simulink model "Flight_Simulation"  (R2021b)
settings: Solver=ode4  StartTime=0.0  StopTime=20  FixedStep=Settings.Simulation.step_size  RelTol=1e-3  EnableMultiTasking=on
undefined symbols (not defined in the file or in its folder): AeroCoeff, Aircraft, ControlGains, dLEF, Environment, F, Light, MIL, Settings, Trim, trim_control, trim_state, trim_thrust
libraries: simulink x19, simulink_extras x14, slpidlib x2, aerolibfltsims x2, aerolibwind2 x1, vrlib x1
(part 1 of 5)
settings Model: Creator=ole_o  LastModifiedBy=s2051295
settings SolverCC: AlgebraicLoopSolver=TrustRegion
settings DataIOCC: Decimation=50  ExternalInput=U_in  InitialState=[]  LoadExternalInput=on  SaveFormat=StructureWithTime  ReturnWorkspaceOutputs=off  TimeSaveName=t_out  OutputSaveName=X_out, X_dot_out, Y_out  SignalLoggingName=sigsOut
settings OptimizationCC: BooleanDataType=off  DefaultParameterBehavior=Inlined  BufferReuse=off
settings DebuggingCC: UnderspecifiedInitializationDetection=Classic  MergeDetectMultiDrivingBlocksExec=none  SignalResolutionControl=TryResolveAllWithWarning  MultiTaskDSMMsg=warning  MultiTaskCondExecSysMsg=none
settings HardwareCC: ProdBitPerPointer=32  ProdBitPerSizeT=32  ProdBitPerPtrDiffT=32  ProdWordSize=32  ProdHWDeviceType=Intel->x86-32 (Windows32)
settings ModelReferenceCC: PropagateSignalLabelsOutOfModel=off
settings SFSimCC: CustomCodeUndefinedFunction=UseInterfaceOnly

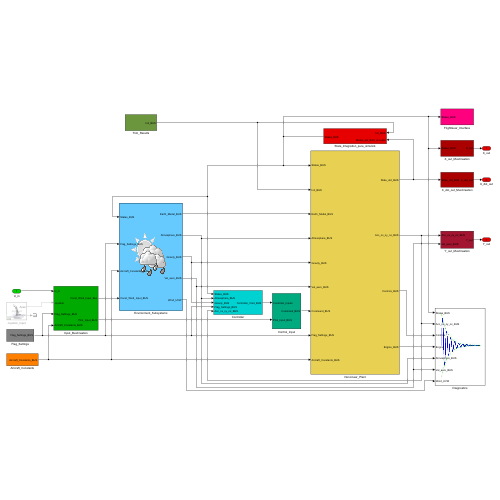
[thumbnail: Simulink's stored preview of the top-level diagram]
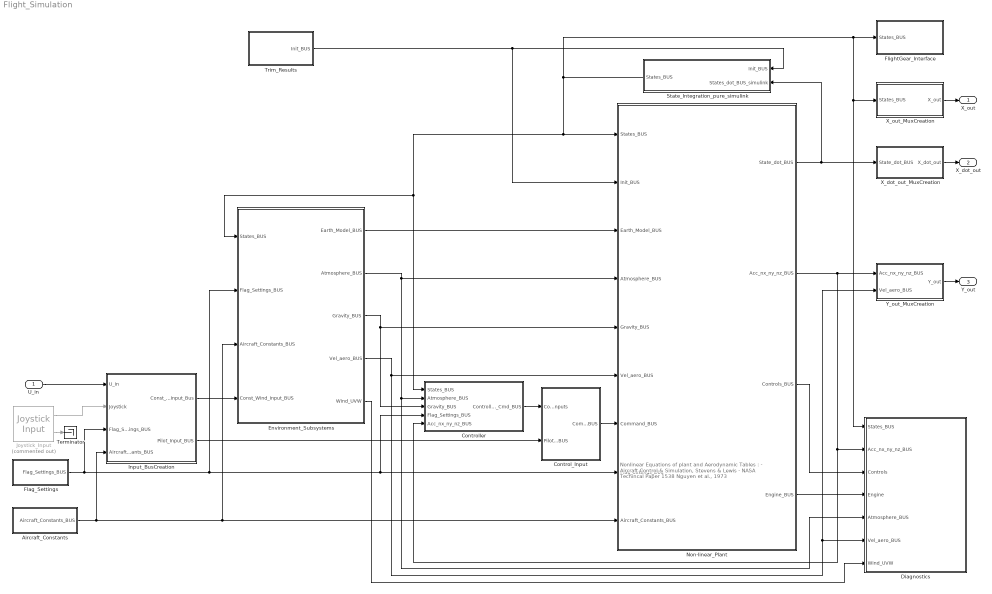
== system Flight_Simulation ==
  note: Nonlinear Equations of plant and Aerodynamic Tables :
      | - Aircraft Control & Simulation, Stevens & Lewis
      | - NASA Techincal Paper 1538 Nguyen et al., 1973
  U_in : Inport  PortDimensions=8
  Aircraft_Constants : Subsystem
  Control_Input : Subsystem
  Controller : Subsystem
  Diagnostics : Subsystem
      mask Display: image('Diagnostics.jpg'); % Use "Edit Image" on toolstrip to change.
  Environment_Subsystems : Subsystem
      mask Display: image('Wetter.jpg'); % Use "Edit Image" on toolstrip to change.
  Flag_Settings : Subsystem
  FlightGear_Interface : Subsystem
  Input_BusCreation : Subsystem
  Joystick_Input : vrlib/Joystick Input  Commented=on  joyid=1  adjustports=off  forcefeed=off
  Non-linear_Plant : Subsystem
  State_Integration_pure_simulink : Subsystem
  Terminator : Terminator
  Trim_Results : Subsystem
  X_dot_out_MuxCreation : Subsystem
  X_out_MuxCreation : Subsystem
  Y_out_MuxCreation : Subsystem
  X_out : Outport
  X_dot_out : Outport  Port=2
  Y_out : Outport  Port=3
  wires:
  Non-linear_Plant/4(Engine_BUS) -> Diagnostics/4(Engine)
  Input_BusCreation/1(Const_Wind_Input_Bus) -> Environment_Subsystems/4(Const_Wind_Input_BUS)
  Joystick_Input/2 -> Terminator/1
  Non-linear_Plant/3(Controls_BUS) -> Diagnostics/3(Controls)
  Environment_Subsystems/3(Gravity_BUS) -> Non-linear_Plant/5(Gravity_BUS), Controller/3(Gravity_BUS)
  Joystick_Input/1 -> Input_BusCreation/2(Joystick)
  Aircraft_Constants/1(Aircraft_Constants_BUS) -> Environment_Subsystems/3(Aircraft_Constants_BUS), Non-linear_Plant/9(Aircraft_Constants_BUS), Input_BusCreation/4(Aircraft_Constants_BUS)
  X_out_MuxCreation/1(X_out) -> X_out/1
  Environment_Subsystems/4(Vel_aero_BUS) -> Non-linear_Plant/6(Vel_aero_BUS), Diagnostics/6(Vel_aero_BUS), Y_out_MuxCreation/2(Vel_aero_BUS)
  Controller/1(Controller_Cmd_BUS) -> Control_Input/1(Controller_Inputs)
  Environment_Subsystems/2(Atmosphere_BUS) -> Non-linear_Plant/4(Atmosphere_BUS), Diagnostics/5(Atmosphere_BUS), Controller/2(Atmosphere_BUS)
  State_Integration_pure_simulink/1(States_BUS) -> FlightGear_Interface/1(States_BUS), X_out_MuxCreation/1(States_BUS), Diagnostics/1(States_BUS), Non-linear_Plant/1(States_BUS), Environment_Subsystems/1(States_BUS), Controller/1(States_BUS)
  Y_out_MuxCreation/1(Y_out) -> Y_out/1
  Input_BusCreation/2(Pilot_Input_BUS) -> Control_Input/2(Pilot_Input_BUS)
  Trim_Results/1(Init_BUS) -> Non-linear_Plant/2(Init_BUS), State_Integration_pure_simulink/1(Init_BUS)
  Control_Input/1(Command_BUS) -> Non-linear_Plant/7(Command_BUS)
  X_dot_out_MuxCreation/1(X_dot_out) -> X_dot_out/1
  Flag_Settings/1(Flag_Settings_BUS) -> Environment_Subsystems/2(Flag_Settings_BUS), Non-linear_Plant/8(Flag_Settings_BUS), Controller/4(Flag_Settings_BUS), Input_BusCreation/3(Flag_Settings_BUS)
  U_in/1 -> Input_BusCreation/1(U_in)
  Non-linear_Plant/1(State_dot_BUS) -> X_dot_out_MuxCreation/1(State_dot_BUS), State_Integration_pure_simulink/2(States_dot_BUS_simulink)
  Non-linear_Plant/2(Acc_nx_ny_nz_BUS) -> Y_out_MuxCreation/1(Acc_nx_ny_nz_BUS), Controller/5(Acc_nx_ny_nz_BUS), Diagnostics/2(Acc_nx_ny_nz_BUS)
  Environment_Subsystems/1(Earth_Model_BUS) -> Non-linear_Plant/3(Earth_Model_BUS)
  Environment_Subsystems/5(Wind_UVW) -> Diagnostics/7(Wind_UVW)

== system Flight_Simulation/Aircraft_Constants ==
  Bus Creator : BusCreator  Inputs=8
  CG_Reference_Location : Subsystem
  Constant : Constant  Value=Aircraft.LandingGearFlg
  Constant1 : Constant  Value=Aircraft.Flaps_degrees
  Constant2 : Constant  Value=Aircraft.F_g.final
  Control_Surface_Model : Subsystem
  Engine_Const : Subsystem
  Mass_Properties : Subsystem
  Wing_Dimensions : Subsystem
  Aircraft_Constants_BUS : Outport
  wires:
  Mass_Properties/1(Mass_Properties_BUS) -> Bus Creator/1
  Wing_Dimensions/1(Wing_Dimension_BUS) -> CG_Reference_Location/1(Wing_Dimension_BUS), Bus Creator/2
  CG_Reference_Location/1(CG_BUS) -> Bus Creator/3
  Engine_Const/1(Engine_Const_BUS) -> Bus Creator/5
  Control_Surface_Model/1(Control_Surface_Const_BUS) -> Bus Creator/4
  Bus Creator/1 -> Aircraft_Constants_BUS/1  "Aircraft_Constants_BUS"
  Constant/1 -> Bus Creator/6  "LandingGearFlg"
  Constant1/1 -> Bus Creator/7  "Flaps_degrees"
  Constant2/1 -> Bus Creator/8  "FlightProfileAlleviationFactor_Fg"

== system Flight_Simulation/Control_Input ==
  Controller_Inputs : Inport
  Pilot_Input_BUS : Inport  Port=2
  Aileron Disturbance : Subsystem
  Bus Creator : BusCreator  Inputs=5
  Bus Selector : BusSelector  OutputSignals=Thrust_N_ctrl,Elevator_deg_ctrl,Aileron_deg_ctrl,Rudder_deg_ctrl,Speedbrakes_%_ctrl
  Bus Selector1 : BusSelector  OutputSignals=Thrust_in_N,Elevator_in_deg,Aileron_in_deg,Rudder_in_deg,Speedbrakes_in_%
  Elevator Disturbance : Subsystem
  Rudder Disturbance : Subsystem
  Sum1 : Sum  Inputs=+++  InputSameDT=on  SaturateOnIntegerOverflow=on  OutDataTypeStr=Inherit: Same as first input
  Sum2 : Sum  Inputs=+++  InputSameDT=on  SaturateOnIntegerOverflow=on  OutDataTypeStr=Inherit: Same as first input
  Sum3 : Sum  Inputs=+++  InputSameDT=on  SaturateOnIntegerOverflow=on  OutDataTypeStr=Inherit: Same as first input
  Sum4 : Sum  Inputs=++|  InputSameDT=on  SaturateOnIntegerOverflow=on  OutDataTypeStr=Inherit: Same as first input
  Sum5 : Sum  Inputs=++|  InputSameDT=on  SaturateOnIntegerOverflow=on  OutDataTypeStr=Inherit: Same as first input
  Command_BUS : Outport
  wires:
  Sum4/1 -> Bus Creator/1  "Thrust_cmd_N"
  Bus Selector/3 -> Sum2/1  "<Aileron_deg_ctrl>"
  Bus Selector/2 -> Sum1/1  "<Elevator_deg_ctrl>"
  Bus Selector/4 -> Sum3/1  "<Rudder_deg_ctrl>"
  Bus Creator/1 -> Command_BUS/1  "Command_BUS"
  Sum1/1 -> Bus Creator/2  "Elevator_cmd_deg"
  Sum2/1 -> Bus Creator/3  "Aileron_cmd_deg"
  Sum3/1 -> Bus Creator/4  "Rudder_cmd_deg"
  Controller_Inputs/1 -> Bus Selector/1
  Bus Selector/1 -> Sum4/1  "<Thrust_N_ctrl>"
  Rudder Disturbance/1(Rudder_Disturbance) -> Sum3/3
  Aileron Disturbance/1(Aileron_Disturbance) -> Sum2/3
  Elevator Disturbance/1(Elevator_Disturbance) -> Sum1/3
  Pilot_Input_BUS/1 -> Bus Selector1/1
  Bus Selector1/1 -> Sum4/2  "<Thrust_in_N>"
  Bus Selector1/2 -> Sum1/2  "<Elevator_in_deg>"
  Bus Selector1/3 -> Sum2/2  "<Aileron_in_deg>"
  Bus Selector1/4 -> Sum3/2  "<Rudder_in_deg>"
  Bus Selector1/5 -> Sum5/2  "<Speedbrakes_in_%>"
  Bus Selector/5 -> Sum5/1  "<Speedbrakes_%_ctrl>"
  Sum5/1 -> Bus Creator/5  "Speedbrakes_cmd_%"

== system Flight_Simulation/Controller ==
  note: must not change name and location
      | - would interfere with TrimAndLin
  States_BUS : Inport
  Atmosphere_BUS : Inport  Port=2
  Gravity_BUS : Inport  Port=3
  Flag_Settings_BUS : Inport  Port=4
  Acc_nx_ny_nz_BUS : Inport  Port=5
  Autopilot : Subsystem
  Bus Creator : BusCreator  Inputs=5
  Bus Selector : BusSelector  OutputSignals=Linearization_Flag,Trim_Flag
  Bypass for TrimAndLin : Switch  Criteria=u2 > Threshold
  Constant{,1..5} (6 alike) : Constant  Value=0
  Logical Operator : Logic  Operator=NOR  AllPortsSameDT=off  OutDataTypeStr=boolean
  Step : Step  Time=0.2  Before=-10  After=0  SampleTime=0
  Terminator : Terminator
  Controller_Cmd_BUS : Outport
  wires:
  States_BUS/1 -> Autopilot/3(States_BUS)
  Constant5/1 -> Bus Creator/2  "Elevator_deg_ctrl"
  Constant/1 -> Bus Creator/1  "Thrust_N_ctrl"
  Constant2/1 -> Bus Creator/3  "Aileron_deg_ctrl"
  Constant3/1 -> Bus Creator/4  "Rudder_deg_ctrl"
  Bus Creator/1 -> Controller_Cmd_BUS/1  "Controller_Cmd_BUS"
  Autopilot/1(d_E) -> Bypass for TrimAndLin/1
  Flag_Settings_BUS/1 -> Bus Selector/1
  Bus Selector/1 -> Logical Operator/1  "<Linearization_Flag>"
  Bus Selector/2 -> Logical Operator/2  "<Trim_Flag>"
  Logical Operator/1 -> Bypass for TrimAndLin/2
  Constant1/1 -> Bypass for TrimAndLin/3  "d_Ec"
  Constant4/1 -> Bus Creator/5  "Speedbrakes_%_ctrl"
  Acc_nx_ny_nz_BUS/1 -> Terminator/1
  Gravity_BUS/1 -> Autopilot/1(Gravity_BUS)
  Atmosphere_BUS/1 -> Autopilot/2(Atmosphere_BUS)

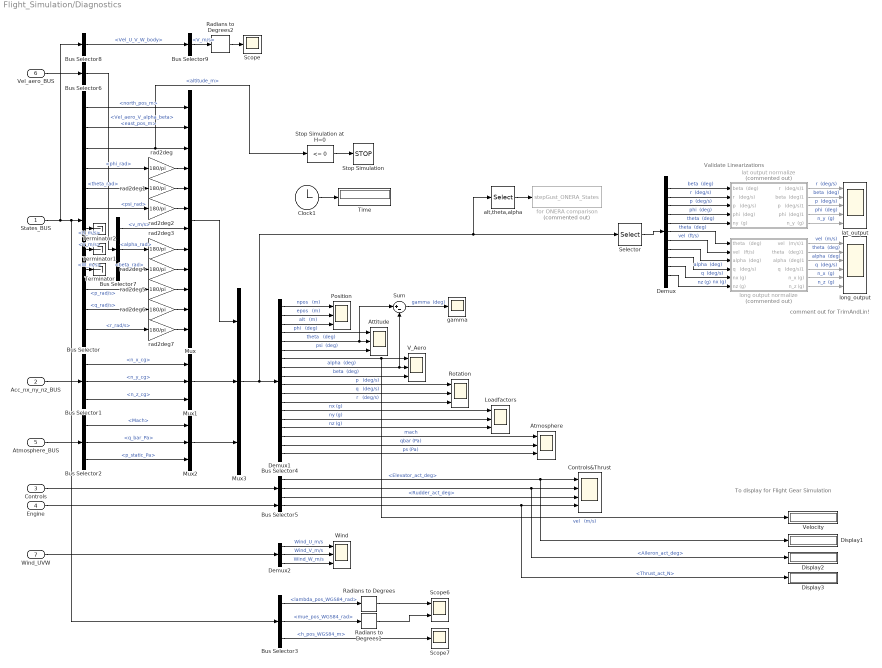
== system Flight_Simulation/Diagnostics ==
  note: To display for
      | Flight Gear Simulation
  note: comment out for TrimAndLin!
  note: Validate Linearizations
  States_BUS : Inport
  Acc_nx_ny_nz_BUS : Inport  Port=2
  Controls : Inport  Port=3
  Engine : Inport  Port=4
  Atmosphere_BUS : Inport  Port=5
  Vel_aero_BUS : Inport  Port=6
  Wind_UVW : Inport  Port=7
  Atmosphere : Scope  NumInputPorts=3
  Attitude : Scope  NumInputPorts=3
  Bus Selector : BusSelector  OutputSignals=Position_north_east_alt.north_pos_m,Position_north_east_alt.east_pos_m,Position_north_east_alt.altitude_m,Angles_phi_theta_psi.phi_rad,Angles_phi_theta_psi.theta_rad,Angles_phi_theta_psi.psi_rad,Vel_U_V_W_body.U_m/s,Vel_U_V_W_body.V_m/s,Vel_U_V_W_body.W_m/s,Rates_p_q_r.p_rad/s,Rates_p_q_r.q_rad/s,Rates_p_q_r.r_rad/s
  Bus Selector1 : BusSelector  OutputSignals=n_x_cg,n_y_cg,n_z_cg
  Bus Selector2 : BusSelector  OutputSignals=Mach,q_bar_Pa,p_static_Pa
  Bus Selector3 : BusSelector  OutputSignals=Pos_WGS84.lambda_pos_WGS84_rad,Pos_WGS84.mue_pos_WGS84_rad,Pos_WGS84.h_pos_WGS84_m
  Bus Selector4 : BusSelector  OutputSignals=Elevator_act_deg,Aileron_act_deg,Rudder_act_deg
  Bus Selector5 : BusSelector  OutputSignals=Thrust_act_N
  Bus Selector6 : BusSelector  OutputSignals=Vel_aero_V_alpha_beta
  Bus Selector7 : BusSelector  OutputSignals=v_m/s,alpha_rad,beta_rad
  Bus Selector8 : BusSelector  OutputSignals=Vel_U_V_W_body
  Bus Selector9 : BusSelector  OutputSignals=V_m/s
  Clock1 : Clock
  Controls&Thrust : Scope  NumInputPorts=4
  Demux : Demux  Outputs=11
  Demux1 : Demux  Outputs=18
      settings: DisplayOption=none
  Demux2 : Demux  Outputs=3
  Display1 : Display
  Display2 : Display
  Display3 : Display
  Loadfactors : Scope  NumInputPorts=3
  Mux : Mux  Inputs=12
  Mux1 : Mux  Inputs=3
  Mux2 : Mux  Inputs=3
  Mux3 : Mux  Inputs=3
  Position : Scope  NumInputPorts=3
  Radians to Degrees : simulink_extras/Transformations/Radians to Degrees
  Radians to Degrees1 : simulink_extras/Transformations/Radians to Degrees
  Radians to Degrees2 : simulink_extras/Transformations/Radians to Degrees
  Rotation : Scope  NumInputPorts=3
  Scope : Scope
  Scope6 : Scope  NumInputPorts=2
  Scope7 : Scope
  Selector : Selector  InputPortWidth=18  IndexOptions=Index vector (dialog)  Indices=[9 12 10 4 14 5 7 8 11 13 15]  OutputSizes=1
  Stop Simulation : Stop
  Stop Simulation at H=0 : simulink/Logic and Bit Operations/Compare To Constant  relop=<=  const=0  OutDataTypeStr=boolean
  Sum : Sum  Inputs=|+-
  Terminator : Terminator
  Terminator1 : Terminator
  Terminator2 : Terminator
  Time : Display
  V_Aero : Scope  NumInputPorts=3
  Velocity : Display
  Wind : Scope  NumInputPorts=3
  alt,theta,alpha : Selector  InputPortWidth=18  IndexOptions=Index vector (dialog)  Indices=[3 5 8]  OutputSizes=1
  for ONERA comparison : ToWorkspace  Commented=on  VariableName=stepGust_ONERA_States  SampleTime=-1
  gamma : Scope
  lat output normalize : Subsystem  Commented=on
  lat_output : Scope  NumInputPorts=5
  long output normalize : Subsystem  Commented=on
  long_output : Scope  NumInputPorts=6
  rad2deg{,1..7} (8 alike) : Gain  Gain=180/pi
  wires:
  Demux1/1 -> Position/1  "npos   (m)"
  Demux1/2 -> Position/2  "epos   (m)"
  Demux1/3 -> Position/3  "alt   (m)"
  Demux1/5 -> Attitude/2, Sum/1  "theta   (deg)"
  Demux1/6 -> Attitude/3  "psi  (deg)"
  Demux1/7 -> V_Aero/1, Velocity/1  "vel   (m/s)"
  Demux1/9 -> V_Aero/3  "beta  (deg)"
  Demux1/10 -> Rotation/1  "p   (deg/s)"
  Demux1/11 -> Rotation/2  "q   (deg/s)"
  Demux1/12 -> Rotation/3  "r   (deg/s)"
  Demux1/13 -> Loadfactors/1  "nx (g)"
  Demux1/14 -> Loadfactors/2  "ny (g)"
  Demux1/15 -> Loadfactors/3  "nz (g)"
  Demux1/4 -> Attitude/1  "phi   (deg)"
  Demux1/16 -> Atmosphere/1  "mach"
  Demux1/17 -> Atmosphere/2  "qbar (Pa)"
  Demux1/18 -> Atmosphere/3  "ps (Pa)"
  States_BUS/1 -> Bus Selector8/1, Bus Selector3/1, Bus Selector/1
  Bus Selector/1 -> Mux/1  "<north_pos_m>"
  Bus Selector/2 -> Mux/2  "<east_pos_m>"
  Bus Selector/11 -> rad2deg6/1  "<q_rad/s>"
  Bus Selector/10 -> rad2deg5/1  "<p_rad/s>"
  Bus Selector/12 -> rad2deg7/1  "<r_rad/s>"
  Bus Selector/4 -> rad2deg/1  "<phi_rad>"
  Bus Selector/3 -> Stop Simulation at H=0/1, Mux/3  "<altitude_m>"
  Bus Selector/5 -> rad2deg1/1  "<theta_rad>"
  Bus Selector/6 -> rad2deg2/1  "<psi_rad>"
  rad2deg/1 -> Mux/4
  rad2deg1/1 -> Mux/5
  rad2deg2/1 -> Mux/6
  rad2deg3/1 -> Mux/8
  rad2deg4/1 -> Mux/9
  rad2deg5/1 -> Mux/10
  rad2deg6/1 -> Mux/11
  rad2deg7/1 -> Mux/12
  Mux/1 -> Mux3/1
  Acc_nx_ny_nz_BUS/1 -> Bus Selector1/1
  Bus Selector1/2 -> Mux1/2  "<n_y_cg>"
  Bus Selector1/1 -> Mux1/1  "<n_x_cg>"
  Bus Selector1/3 -> Mux1/3  "<n_z_cg>"
  Atmosphere_BUS/1 -> Bus Selector2/1
  Bus Selector2/3 -> Mux2/3  "<p_static_Pa>"
  Bus Selector2/2 -> Mux2/2  "<q_bar_Pa>"
  Bus Selector2/1 -> Mux2/1  "<Mach>"
  Mux2/1 -> Mux3/3
  Mux1/1 -> Mux3/2
  Mux3/1 -> alt,theta,alpha/1, Selector/1, Demux1/1
  Bus Selector3/1 -> Radians to Degrees/1  "<lambda_pos_WGS84_rad>"
  Bus Selector3/2 -> Radians to Degrees1/1  "<mue_pos_WGS84_rad>"
  Bus Selector3/3 -> Scope7/1  "<h_pos_WGS84_m>"
  Radians to Degrees1/1 -> Scope6/2
  Radians to Degrees/1 -> Scope6/1
  Clock1/1 -> Time/1
  long output normalize/1(vel   (m/s)1) -> long_output/1  "vel  (m/s)"
  long output normalize/2(theta   (deg)1) -> long_output/2  "theta  (deg)"
  long output normalize/3(alpha  (deg)1) -> long_output/3  "alpha  (deg)"
  long output normalize/6(n_z (g)) -> long_output/6  "n_z  (g)"
  Sum/1 -> gamma/1  "gamma  (deg)"
  Demux1/8 -> V_Aero/2, Sum/2  "alpha  (deg)"
  Controls/1 -> Bus Selector4/1
  Bus Selector4/1 -> Display1/1, Controls&Thrust/1  "<Elevator_act_deg>"
  Bus Selector4/2 -> Display2/1, Controls&Thrust/2  "<Aileron_act_deg>"
  Bus Selector5/1 -> Controls&Thrust/4, Display3/1  "<Thrust_act_N>"
  Engine/1 -> Bus Selector5/1
  long output normalize/4(q   (deg/s)1) -> long_output/4  "q  (deg/s)"
  lat output normalize/2(beta  (deg)1) -> lat_output/2  "beta  (deg)"
  lat output normalize/1(r   (deg/s)1) -> lat_output/1  "r  (deg/s)"
  lat output normalize/3(p   (deg/s)1) -> lat_output/3  "p  (deg/s)"
  lat output normalize/4(phi  (deg)1) -> lat_output/4  "phi  (deg)"
  Selector/1 -> Demux/1
  Demux/2 -> lat output normalize/2(r   (deg/s))  "r  (deg/s)"
  Demux/3 -> lat output normalize/3(p   (deg/s))  "p  (deg/s)"
  Demux/4 -> lat output normalize/4(phi  (deg))  "phi  (deg)"
  Demux/6 -> long output normalize/1(theta   (deg))  "theta  (deg)"
  Demux/7 -> long output normalize/2(vel   (ft/s))  "vel  (ft/s)"
  Demux/8 -> long output normalize/3(alpha  (deg))  "alpha  (deg)"
  Demux/9 -> long output normalize/4(q   (deg/s))  "q  (deg/s)"
  Demux/11 -> long output normalize/6(nz (g))  "nz (g)"
  Demux/1 -> lat output normalize/1(beta  (deg))  "beta  (deg)"
  Bus Selector4/3 -> Controls&Thrust/3  "<Rudder_act_deg>"
  Stop Simulation at H=0/1 -> Stop Simulation/1
  Wind_UVW/1 -> Demux2/1
  Demux2/1 -> Wind/1  "Wind_U_m/s"
  Demux2/2 -> Wind/2  "Wind_V_m/s"
  Demux2/3 -> Wind/3  "Wind_W_m/s"
  alt,theta,alpha/1 -> for ONERA comparison/1
  Vel_aero_BUS/1 -> Bus Selector6/1
  Bus Selector6/1 -> Bus Selector7/1  "<Vel_aero_V_alpha_beta>"
  Bus Selector7/2 -> rad2deg3/1  "<alpha_rad>"
  Bus Selector7/3 -> rad2deg4/1  "<beta_rad>"
  Demux/10 -> long output normalize/5(nx (g))  "nx (g)"
  long output normalize/5(n_x (g)) -> long_output/5  "n_x  (g)"
  Demux/5 -> lat output normalize/5(ny  (g))  "theta  (deg)"
  lat output normalize/5(n_y  (g)) -> lat_output/5  "n_y  (g)"
  Bus Selector7/1 -> Mux/7  "<v_m/s>"
  Bus Selector/9 -> Terminator/1  "<W_m/s>"
  Bus Selector/7 -> Terminator2/1  "<U_m/s>"
  Bus Selector/8 -> Terminator1/1  "<V_m/s>"
  Bus Selector8/1 -> Bus Selector9/1  "<Vel_U_V_W_body>"
  Bus Selector9/1 -> Radians to Degrees2/1  "<V_m/s>"
  Radians to Degrees2/1 -> Scope/1

== system Flight_Simulation/Environment_Subsystems ==
  note: more efficient
  note: must not change name and location
      | - would interfere with TrimAndLin
  States_BUS : Inport
  Flag_Settings_BUS : Inport  Port=2
  Aircraft_Constants_BUS : Inport  Port=3
  Const_Wind_Input_BUS : Inport  Port=4
  Earth_Model : Subsystem
  Gravity_Model_simple : Subsystem
  ISA_StandardAtmosphere_Model_ScriptVersion : Subsystem
  ISA_StandardAtmosphere_Model_SimulinkVersion : Subsystem
  Manual Switch : ManualSwitch
  Wind_Input : Subsystem
  Wind_Model : Subsystem
  Earth_Model_BUS : Outport
  Atmosphere_BUS : Outport  Port=2
  Gravity_BUS : Outport  Port=3
  Vel_aero_BUS : Outport  Port=4
  Wind_UVW : Outport  Port=5
  wires:
  Gravity_Model_simple/1(Gravity_BUS) -> ISA_StandardAtmosphere_Model_SimulinkVersion/2(Gravity_BUS), ISA_StandardAtmosphere_Model_ScriptVersion/2(Gravity_BUS), Gravity_BUS/1
  Earth_Model/1(Earth_Model_BUS) -> Earth_Model_BUS/1
  Aircraft_Constants_BUS/1 -> Wind_Model/3(Aircraft_Constants_BUS)
  States_BUS/1 -> Wind_Model/2(States_BUS), Wind_Input/1(States_BUS), ISA_StandardAtmosphere_Model_SimulinkVersion/1(States_BUS), ISA_StandardAtmosphere_Model_ScriptVersion/1(States_BUS), Gravity_Model_simple/1(States_BUS), Earth_Model/1(States_BUS)
  ISA_StandardAtmosphere_Model_ScriptVersion/1(Atmosphere_BUS) -> Manual Switch/1
  ISA_StandardAtmosphere_Model_SimulinkVersion/1(Atmosphere_BUS) -> Manual Switch/2
  Manual Switch/1 -> Atmosphere_BUS/1, Wind_Model/1(Atmosphere_BUS)  "Atmosphere_BUS"
  Wind_Model/1(Wind_BUS) -> Wind_UVW/1, Wind_Input/2(Wind_BUS)  "Wind_Vel_UVWe_m/s"
  Const_Wind_Input_BUS/1 -> Wind_Input/4(Const_Wind_Vel_UVWe_m/s)  "Const_Wind_Vel_UVWe_m/s"
  Flag_Settings_BUS/1 -> Wind_Input/3(Flag_Settings_BUS)  "Flag_Settings_BUS"
  Wind_Input/1(Vel_aero_BUS) -> ISA_StandardAtmosphere_Model_SimulinkVersion/3(Vel_aero_BUS), ISA_StandardAtmosphere_Model_ScriptVersion/3(Vel_Aero_BUS), Vel_aero_BUS/1

== system Flight_Simulation/Flag_Settings ==
  Bus Creator : BusCreator  Inputs=3
  Fidelity_Flag : Constant  Value=0
  Lin_Flag : Constant  Value=0
  Trim_Flag : Constant  Value=0
  Flag_Settings_BUS : Outport
  wires:
  Fidelity_Flag/1 -> Bus Creator/1  "Fidelity_Flag"
  Bus Creator/1 -> Flag_Settings_BUS/1  "Flag_Settings_BUS"
  Lin_Flag/1 -> Bus Creator/2  "Linearization_Flag"
  Trim_Flag/1 -> Bus Creator/3  "Trim_Flag"

== system Flight_Simulation/FlightGear_Interface ==
  note: Remark: Set correct Flight Gear installation path
  note: don't rename
      | or IP-address cannot automatically be set
  States_BUS : Inport
  Bus Selector2 : BusSelector  OutputSignals=Angles_phi_theta_psi
  Bus Selector3 : BusSelector  OutputSignals=phi_rad,theta_rad,psi_rad
  Bus Selector4 : BusSelector  OutputSignals=Pos_WGS84
  Bus Selector5 : BusSelector  OutputSignals=lambda_pos_WGS84_rad,mue_pos_WGS84_rad,h_pos_WGS84_m
  Display : Display
  Display1 : Display
  Display2 : Display
  FG_simpleInterface : aerolibfltsims/FlightGear Preconfigured 6DoF Animation  Commented=on  xFlightGearVersion=v2019.1  DestinationIpAddress=192.168.0.166  DestinationPort=5502  SampleTime=-1  packetVersion=24
  GenerateRunScript : aerolibfltsims/Generate Run Script  Architecture=Win64  dataFlow=Receive  GeometryModelName=c172p  AirportId=EDDC  RunwayId=22  InitialAltitude=15000  InitialHeading=113  OffsetDistance=4.72  OffsetAzimuth=0  InstallScenery=on  DisableShaders=off  OriginAddress=127.0.0.1  DestinationPort=5502  OriginPort=5502  LocalAddress=192.168.0.166  OutputFileName=runfg.bat  FlightGearBaseDirectory=D:\FlightGear 2020.3
  Mux1 : Mux  Inputs=6
  Radians to Degrees : simulink_extras/Transformations/Radians to Degrees
  Radians to Degrees1 : simulink_extras/Transformations/Radians to Degrees
  wires:
  States_BUS/1 -> Bus Selector2/1, Bus Selector4/1
  Bus Selector2/1 -> Bus Selector3/1  "<Angles_phi_theta_psi>"
  Bus Selector3/1 -> Mux1/4  "<phi_rad>"
  Bus Selector3/2 -> Mux1/5  "<theta_rad>"
  Bus Selector3/3 -> Mux1/6  "<psi_rad>"
  Mux1/1 -> FG_simpleInterface/1
  Bus Selector4/1 -> Bus Selector5/1  "<Pos_WGS84>"
  Bus Selector5/1 -> Radians to Degrees/1  "<lambda_pos_WGS84_rad>"
  Bus Selector5/2 -> Radians to Degrees1/1  "<mue_pos_WGS84_rad>"
  Bus Selector5/3 -> Display2/1, Mux1/3  "<h_pos_WGS84_m>"
  Radians to Degrees/1 -> Mux1/1, Display/1
  Radians to Degrees1/1 -> Display1/1, Mux1/2

== system Flight_Simulation/Input_BusCreation ==
  U_in : Inport
  Joystick : Inport  Port=2
  Flag_Settings_BUS : Inport  Port=3
  Aircraft_Constants_BUS : Inport  Port=4
  Aileron : Display
  Bus Creator : BusCreator  Inputs=3
  Bus Creator1 : BusCreator  Inputs=5
  Demux : Demux  Outputs=8
  Elevator : Display
  Evaluate Joystick Input : Subsystem
  JS_Aileron : Display
  JS_Elevator : Display
  JS_Thrust : Display
  Manual Switch : ManualSwitch  CurrentSetting=0
  Sum : Sum  Inputs=++|
  Sum1 : Sum  Inputs=++|
  Thrust : Display
  Const_Wind_Input_Bus : Outport
  Pilot_Input_BUS : Outport  Port=2
  wires:
  U_in/1 -> Demux/1
  Evaluate Joystick Input/3(Joystick_Thrust_N) -> Manual Switch/1, JS_Thrust/1  "Thrust_in_N"
  Sum1/1 -> Aileron/1, Bus Creator1/3  "Aileron_in_deg"
  Bus Creator1/1 -> Pilot_Input_BUS/1  "Pilot_Input_BUS"
  Demux/4 -> Bus Creator1/4  "Rudder_in_deg"
  Sum/1 -> Elevator/1, Bus Creator1/2  "Elevator_in_deg"
  Demux/6 -> Bus Creator/1  "const_u_wind_m/s"
  Bus Creator/1 -> Const_Wind_Input_Bus/1  "Wind_Vel_UVW_m/s"
  Demux/7 -> Bus Creator/2  "const_v_wind_m/s"
  Demux/8 -> Bus Creator/3  "const_w_wind_m/s"
  Aircraft_Constants_BUS/1 -> Evaluate Joystick Input/1(Aircraft_Constants_BUS)
  Flag_Settings_BUS/1 -> Evaluate Joystick Input/2(Flag_Settings_BUS)
  Joystick/1 -> Evaluate Joystick Input/3(Joystick)
  Evaluate Joystick Input/1(Joystick_Aileron_deg) -> Sum1/1, JS_Aileron/1
  Evaluate Joystick Input/2(Joystick_Elevator_deg) -> Sum/1, JS_Elevator/1
  Demux/2 -> Sum/2  "Elevator_in_deg"
  Demux/3 -> Sum1/2  "Aileron_in_deg"
  Manual Switch/1 -> Thrust/1, Bus Creator1/1  "Thrust_in_N"
  Demux/1 -> Manual Switch/2  "Thrust_in_N"
  Demux/5 -> Bus Creator1/5  "Speedbrakes_in_%"

== system Flight_Simulation/Non-linear_Plant ==
  States_BUS : Inport
  Init_BUS : Inport  Port=2
  Earth_Model_BUS : Inport  Port=3
  Atmosphere_BUS : Inport  Port=4
  Gravity_BUS : Inport  Port=5
  Vel_aero_BUS : Inport  Port=6
  Command_BUS : Inport  Port=7
  Flag_Settings_BUS : Inport  Port=8
  Aircraft_Constants_BUS : Inport  Port=9
  6DOF_Equations : Subsystem
      mask Display: image('Flightdynamics.png'); % Use "Edit Image" on toolstrip to change.
  Actuator_Models : Subsystem
  Aerodynamic_Modul : Subsystem
  Engine_Model : Subsystem
  State_dot_BUS : Outport
  Acc_nx_ny_nz_BUS : Outport  Port=2
  Controls_BUS : Outport  Port=3
  Engine_BUS : Outport  Port=4
  wires:
  Flag_Settings_BUS/1 -> Engine_Model/2(Flag_Settings_BUS), Actuator_Models/3(Flag_Settings_BUS)
  Command_BUS/1 -> Engine_Model/1(Command_BUS), Actuator_Models/2(Command_BUS)
  Aircraft_Constants_BUS/1 -> Aerodynamic_Modul/4(Aircraft_Constant_BUS), Actuator_Models/5(Aircraft_Constants_BUS), Engine_Model/4(Aircraft_Constants_BUS), 6DOF_Equations/5(Aircraft_Constants_BUS)
  Engine_Model/1(Engine_BUS) -> Engine_BUS/1, Aerodynamic_Modul/7(Engine_BUS), 6DOF_Equations/4(Engine_BUS)
  Atmosphere_BUS/1 -> Engine_Model/5(Atmosphere_BUS), Actuator_Models/6(Atmosphere_BUS), Aerodynamic_Modul/1(Atmosphere_BUS)
  Gravity_BUS/1 -> 6DOF_Equations/6(Gravity_BUS)
  States_BUS/1 -> Aerodynamic_Modul/2(States_BUS), 6DOF_Equations/1(States_BUS)
  Init_BUS/1 -> Engine_Model/3(Init_BUS), Actuator_Models/4(Init_BUS)
  Earth_Model_BUS/1 -> 6DOF_Equations/7(Earth_Model_BUS)
  Actuator_Models/1(Flaps_BUS) -> Aerodynamic_Modul/5(LE_Flaps_BUS)
  Actuator_Models/2(Controls_BUS) -> Controls_BUS/1, Aerodynamic_Modul/6(Controls_BUS)
  6DOF_Equations/1(State_dot_BUS) -> State_dot_BUS/1
  Aerodynamic_Modul/1(Forces_total_BUS) -> 6DOF_Equations/2(AeroForces_total_BUS)
  Aerodynamic_Modul/2(Moments_total_BUS) -> 6DOF_Equations/3(AeroMoments_total_BUS)
  6DOF_Equations/2(Acc_nx_ny_nz_BUS) -> Acc_nx_ny_nz_BUS/1
  Vel_aero_BUS/1 -> Actuator_Models/1(Vel_aero_BUS), Aerodynamic_Modul/3(Vel_aero_BUS)

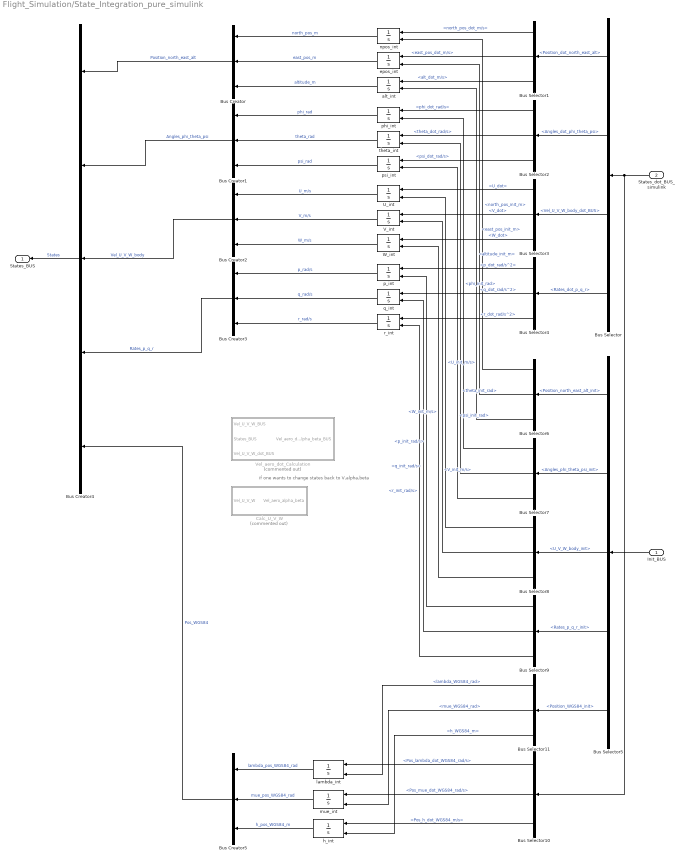
== system Flight_Simulation/State_Integration_pure_simulink ==
  note: if one wants to change states back to V,alpha,beta
  Init_BUS : Inport
  States_dot_BUS_simulink : Inport  Port=2
  Bus Creator{,1..3,5} (5 alike) : BusCreator  Inputs=3
  Bus Creator4 : BusCreator  Inputs=5
  Bus Selector : BusSelector  OutputSignals=Position_dot_BUS.Position_dot_north_east_alt,Angles_dot_phi_theta_psi,Vel_U_V_W_body_dot_BUS,Rates_dot_p_q_r
  Bus Selector1 : BusSelector  OutputSignals=north_pos_dot_m/s,east_pos_dot_m/s,alt_dot_m/s
  Bus Selector10 : BusSelector  OutputSignals=Position_dot_BUS.Pos_WGS84_dot_BUS.Pos_lambda_dot_WGS84_rad/s,Position_dot_BUS.Pos_WGS84_dot_BUS.Pos_mue_dot_WGS84_rad/s,Position_dot_BUS.Pos_WGS84_dot_BUS.Pos_h_dot_WGS84_m/s
  Bus Selector11 : BusSelector  OutputSignals=lambda_WGS84_rad,mue_WGS84_rad,h_WGS84_m
  Bus Selector2 : BusSelector  OutputSignals=phi_dot_rad/s,theta_dot_rad/s,psi_dot_rad/s
  Bus Selector3 : BusSelector  OutputSignals=U_dot,V_dot,W_dot
  Bus Selector4 : BusSelector  OutputSignals=p_dot_rad/s^2,q_dot_rad/s^2,r_dot_rad/s^2
  Bus Selector5 : BusSelector  OutputSignals=X_init_BUS.Position_north_east_alt_init,X_init_BUS.Angles_phi_theta_psi_init,X_init_BUS.U_V_W_body_init,X_init_BUS.Rates_p_q_r_init,X_init_BUS.Position_WGS84_init
  Bus Selector6 : BusSelector  OutputSignals=north_pos_init_m,east_pos_init_m,altitude_init_m
  Bus Selector7 : BusSelector  OutputSignals=phi_init_rad,theta_init_rad,psi_init_rad
  Bus Selector8 : BusSelector  OutputSignals=U_init_m/s,V_init_m/s,W_init_m/s
  Bus Selector9 : BusSelector  OutputSignals=p_init_rad/s,q_init_rad/s,r_init_rad/s
  Calc_U_V_W : Subsystem  Commented=on
  U_int : Integrator  InitialConditionSource=external  InitialCondition=trim_state(7)
  V_int : Integrator  InitialConditionSource=external  InitialCondition=trim_state(8)
  Vel_aero_dot_Calculation : Subsystem  Commented=on
  W_int : Integrator  InitialConditionSource=external  InitialCondition=trim_state(9)
  alt_int : Integrator  InitialConditionSource=external  InitialCondition=trim_state(3)
  epos_int : Integrator  InitialConditionSource=external  InitialCondition=trim_state(2)
  h_int : Integrator  InitialConditionSource=external
  lambda_int : Integrator  InitialConditionSource=external
  mue_int : Integrator  InitialConditionSource=external
  npos_int : Integrator  InitialConditionSource=external  InitialCondition=trim_state(1)
  p_int : Integrator  InitialConditionSource=external  InitialCondition=trim_state(10)
  phi_int : Integrator  InitialConditionSource=external  InitialCondition=trim_state(4)
  psi_int : Integrator  InitialConditionSource=external  InitialCondition=trim_state(6)
  q_int : Integrator  InitialConditionSource=external  InitialCondition=trim_state(11)
  r_int : Integrator  InitialConditionSource=external  InitialCondition=trim_state(12)
  theta_int : Integrator  InitialConditionSource=external  InitialCondition=trim_state(5)
  States_BUS : Outport
  wires:
  U_int/1 -> Bus Creator2/1  "U_m/s"
  Bus Creator4/1 -> States_BUS/1  "States"
  Bus Creator3/1 -> Bus Creator4/4  "Rates_p_q_r"
  q_int/1 -> Bus Creator3/2  "q_rad/s"
  r_int/1 -> Bus Creator3/3  "r_rad/s"
  p_int/1 -> Bus Creator3/1  "p_rad/s"
  Bus Selector4/3 -> r_int/1  "<r_dot_rad/s^2>"
  Bus Selector4/2 -> q_int/1  "<q_dot_rad/s^2>"
  Bus Selector4/1 -> p_int/1  "<p_dot_rad/s^2>"
  Bus Selector/4 -> Bus Selector4/1  "<Rates_dot_p_q_r>"
  Bus Creator2/1 -> Bus Creator4/3  "Vel_U_V_W_body"
  V_int/1 -> Bus Creator2/2  "V_m/s"
  W_int/1 -> Bus Creator2/3  "W_m/s"
  Bus Selector3/3 -> W_int/1  "<W_dot>"
  Bus Selector3/2 -> V_int/1  "<V_dot>"
  Bus Selector3/1 -> U_int/1  "<U_dot>"
  Bus Selector/3 -> Bus Selector3/1  "<Vel_U_V_W_body_dot_BUS>"
  Bus Creator1/1 -> Bus Creator4/2  "Angles_phi_theta_psi"
  phi_int/1 -> Bus Creator1/1  "phi_rad"
  theta_int/1 -> Bus Creator1/2  "theta_rad"
  psi_int/1 -> Bus Creator1/3  "psi_rad"
  Bus Selector2/3 -> psi_int/1  "<psi_dot_rad/s>"
  Bus Selector2/2 -> theta_int/1  "<theta_dot_rad/s>"
  Bus Selector2/1 -> phi_int/1  "<phi_dot_rad/s>"
  Bus Selector/2 -> Bus Selector2/1  "<Angles_dot_phi_theta_psi>"
  Bus Creator/1 -> Bus Creator4/1  "Position_north_east_alt"
  alt_int/1 -> Bus Creator/3  "altitude_m"
  epos_int/1 -> Bus Creator/2  "east_pos_m"
  npos_int/1 -> Bus Creator/1  "north_pos_m"
  Bus Selector1/3 -> alt_int/1  "<alt_dot_m/s>"
  Bus Selector1/2 -> epos_int/1  "<east_pos_dot_m/s>"
  Bus Selector1/1 -> npos_int/1  "<north_pos_dot_m/s>"
  Bus Selector/1 -> Bus Selector1/1  "<Position_dot_north_east_alt>"
  States_dot_BUS_simulink/1 -> Bus Selector10/1, Bus Selector/1
  Init_BUS/1 -> Bus Selector5/1
  Bus Selector9/3 -> r_int/2  "<r_init_rad/s>"
  Bus Selector9/2 -> q_int/2  "<q_init_rad/s>"
  Bus Selector9/1 -> p_int/2  "<p_init_rad/s>"
  Bus Selector5/4 -> Bus Selector9/1  "<Rates_p_q_r_init>"
  Bus Selector8/3 -> W_int/2  "<W_init_m/s>"
  Bus Selector8/2 -> V_int/2  "<V_init_m/s>"
  Bus Selector8/1 -> U_int/2  "<U_init_m/s>"
  Bus Selector5/3 -> Bus Selector8/1  "<U_V_W_body_init>"
  Bus Selector7/3 -> psi_int/2  "<psi_init_rad>"
  Bus Selector7/2 -> theta_int/2  "<theta_init_rad>"
  Bus Selector7/1 -> phi_int/2  "<phi_init_rad>"
  Bus Selector5/2 -> Bus Selector7/1  "<Angles_phi_theta_psi_init>"
  Bus Selector6/3 -> alt_int/2  "<altitude_init_m>"
  Bus Selector6/2 -> epos_int/2  "<east_pos_init_m>"
  Bus Selector6/1 -> npos_int/2  "<north_pos_init_m>"
  Bus Selector5/1 -> Bus Selector6/1  "<Position_north_east_alt_init>"
  Bus Selector10/3 -> h_int/1  "<Pos_h_dot_WGS84_m/s>"
  Bus Selector10/2 -> mue_int/1  "<Pos_mue_dot_WGS84_rad/s>"
  Bus Selector10/1 -> lambda_int/1  "<Pos_lambda_dot_WGS84_rad/s>"
  mue_int/1 -> Bus Creator5/2  "mue_pos_WGS84_rad"
  lambda_int/1 -> Bus Creator5/1  "lambda_pos_WGS84_rad"
  h_int/1 -> Bus Creator5/3  "h_pos_WGS84_m"
  Bus Creator5/1 -> Bus Creator4/5  "Pos_WGS84"
  Bus Selector5/5 -> Bus Selector11/1  "<Position_WGS84_init>"
  Bus Selector11/1 -> lambda_int/2  "<lambda_WGS84_rad>"
  Bus Selector11/2 -> mue_int/2  "<mue_WGS84_rad>"
  Bus Selector11/3 -> h_int/2  "<h_WGS84_m>"

== system Flight_Simulation/Trim_Results ==
  Bus Creator : BusCreator  Inputs=2
  U_init_BusCreation : Subsystem
  X_init_BusCreation : Subsystem
  Init_BUS : Outport
  wires:
  X_init_BusCreation/1(X_init_BUS) -> Bus Creator/1
  U_init_BusCreation/1(U_init_BUS) -> Bus Creator/2
  Bus Creator/1 -> Init_BUS/1

== system Flight_Simulation/X_dot_out_MuxCreation ==
  State_dot_BUS : Inport
  Bus Selector : BusSelector  OutputSignals=Position_dot_BUS.Position_dot_north_east_alt,Angles_dot_phi_theta_psi,Vel_U_V_W_body_dot_BUS,Rates_dot_p_q_r
  Bus Selector1 : BusSelector  OutputSignals=north_pos_dot_m/s,east_pos_dot_m/s,alt_dot_m/s
  Bus Selector2 : BusSelector  OutputSignals=phi_dot_rad/s,theta_dot_rad/s,psi_dot_rad/s
  Bus Selector3 : BusSelector  OutputSignals=U_dot,V_dot,W_dot
  Bus Selector4 : BusSelector  OutputSignals=p_dot_rad/s^2,q_dot_rad/s^2,r_dot_rad/s^2
  Mux : Mux  Inputs=12
  X_dot_out : Outport
  wires:
  State_dot_BUS/1 -> Bus Selector/1
  Bus Selector/1 -> Bus Selector1/1  "<Position_dot_north_east_alt>"
  Bus Selector/2 -> Bus Selector2/1  "<Angles_dot_phi_theta_psi>"
  Bus Selector/3 -> Bus Selector3/1  "<Vel_U_V_W_body_dot_BUS>"
  Bus Selector/4 -> Bus Selector4/1  "<Rates_dot_p_q_r>"
  Bus Selector1/1 -> Mux/1  "<north_pos_dot_m/s>"
  Bus Selector1/2 -> Mux/2  "<east_pos_dot_m/s>"
  Bus Selector1/3 -> Mux/3  "<alt_dot_m/s>"
  Bus Selector2/1 -> Mux/4  "<phi_dot_rad/s>"
  Bus Selector2/2 -> Mux/5  "<theta_dot_rad/s>"
  Bus Selector2/3 -> Mux/6  "<psi_dot_rad/s>"
  Bus Selector3/1 -> Mux/7  "<U_dot>"
  Bus Selector3/2 -> Mux/8  "<V_dot>"
  Bus Selector3/3 -> Mux/9  "<W_dot>"
  Bus Selector4/2 -> Mux/11  "<q_dot_rad/s^2>"
  Bus Selector4/3 -> Mux/12  "<r_dot_rad/s^2>"
  Bus Selector4/1 -> Mux/10  "<p_dot_rad/s^2>"
  Mux/1 -> X_dot_out/1

== system Flight_Simulation/X_out_MuxCreation ==
  States_BUS : Inport
  Bus Selector : BusSelector  OutputSignals=Position_north_east_alt,Angles_phi_theta_psi,Vel_U_V_W_body,Rates_p_q_r
  Bus Selector1 : BusSelector  OutputSignals=north_pos_m,east_pos_m,altitude_m
  Bus Selector2 : BusSelector  OutputSignals=phi_rad,theta_rad,psi_rad
  Bus Selector3 : BusSelector  OutputSignals=U_m/s,V_m/s,W_m/s
  Bus Selector4 : BusSelector  OutputSignals=p_rad/s,q_rad/s,r_rad/s
  Mux : Mux  Inputs=12
  X_out : Outport
  wires:
  Bus Selector4/2 -> Mux/11  "<q_rad/s>"
  Bus Selector4/1 -> Mux/10  "<p_rad/s>"
  Bus Selector3/2 -> Mux/8  "<V_m/s>"
  Bus Selector4/3 -> Mux/12  "<r_rad/s>"
  Bus Selector/2 -> Bus Selector2/1  "<Angles_phi_theta_psi>"
  Bus Selector1/2 -> Mux/2  "<east_pos_m>"
  Mux/1 -> X_out/1  "X_out"
  Bus Selector/3 -> Bus Selector3/1  "<Vel_U_V_W_body>"
  Bus Selector/1 -> Bus Selector1/1  "<Position_north_east_alt>"
  Bus Selector1/3 -> Mux/3  "<altitude_m>"
  Bus Selector2/3 -> Mux/6  "<psi_rad>"
  Bus Selector3/3 -> Mux/9  "<W_m/s>"
  Bus Selector2/2 -> Mux/5  "<theta_rad>"
  Bus Selector1/1 -> Mux/1  "<north_pos_m>"
  Bus Selector/4 -> Bus Selector4/1  "<Rates_p_q_r>"
  Bus Selector3/1 -> Mux/7  "<U_m/s>"
  Bus Selector2/1 -> Mux/4  "<phi_rad>"
  States_BUS/1 -> Bus Selector/1

== system Flight_Simulation/Y_out_MuxCreation ==
  Acc_nx_ny_nz_BUS : Inport
  Vel_aero_BUS : Inport  Port=2
  Bus Selector : BusSelector  OutputSignals=n_x_cg,n_y_cg,n_z_cg
  Bus Selector1 : BusSelector  OutputSignals=Vel_aero_V_alpha_beta.v_m/s,Vel_aero_V_alpha_beta.alpha_rad,Vel_aero_V_alpha_beta.beta_rad
  Mux : Mux  Inputs=6
  Y_out : Outport
  wires:
  Acc_nx_ny_nz_BUS/1 -> Bus Selector/1
  Bus Selector/1 -> Mux/1  "<n_x_cg>"
  Bus Selector/2 -> Mux/2  "<n_y_cg>"
  Bus Selector/3 -> Mux/3  "<n_z_cg>"
  Mux/1 -> Y_out/1
  Vel_aero_BUS/1 -> Bus Selector1/1
  Bus Selector1/1 -> Mux/4  "<v_m/s>"
  Bus Selector1/2 -> Mux/5  "<alpha_rad>"
  Bus Selector1/3 -> Mux/6  "<beta_rad>"

== system Flight_Simulation/Aircraft_Constants/CG_Reference_Location ==
  note: actual center of gravity as a fraction of MAC
  note: reference center of gravity as a fraction of MAC
  Wing_Dimension_BUS : Inport
  Bus Creator : BusCreator  Inputs=3
  Bus Selector : BusSelector  OutputSignals=MAC_m
  Product : Product
  cg : Constant  Value=Aircraft.Dimensions.cg
  cg_ref : Constant  Value=Aircraft.Dimensions.cg_ref
  CG_BUS : Outport
  wires:
  Wing_Dimension_BUS/1 -> Bus Selector/1
  Bus Selector/1 -> Product/1  "<MAC_m>"
  Product/1 -> Bus Creator/1  "X_cg_m"
  cg_ref/1 -> Product/2, Bus Creator/2  "cg_ref_rel"
  Bus Creator/1 -> CG_BUS/1  "cg_BUS"
  cg/1 -> Bus Creator/3  "cg_rel"

== system Flight_Simulation/Aircraft_Constants/Control_Surface_Model ==
  Ail_lag : Constant  Value=Aircraft.Controls.Ail_lag
  Ail_pos_max : Constant  Value=Aircraft.Controls.Ail_pos_max
  Ail_pos_min : Constant  Value=Aircraft.Controls.Ail_pos_min
  Ail_rate_max : Constant  Value=Aircraft.Controls.Ail_rate_max
  Ail_rate_min : Constant  Value=Aircraft.Controls.Ail_rate_min
  Bus Creator : BusCreator  Inputs=3
  Bus Creator1 : BusCreator  Inputs=5
  Bus Creator2 : BusCreator  Inputs=5
  Bus Creator3 : BusCreator  Inputs=5
  Elev_lag : Constant  Value=Aircraft.Controls.Elev_lag
  Elev_pos_max : Constant  Value=Aircraft.Controls.Elev_pos_max
  Elev_pos_min : Constant  Value=Aircraft.Controls.Elev_pos_min
  Elev_rate_max : Constant  Value=Aircraft.Controls.Elev_rate_max
  Elev_rate_min : Constant  Value=Aircraft.Controls.Elev_rate_min
  Rud_lag : Constant  Value=Aircraft.Controls.Rud_lag
  Rud_pos_max : Constant  Value=Aircraft.Controls.Rud_pos_max
  Rud_pos_min : Constant  Value=Aircraft.Controls.Rud_pos_min
  Rud_rate_max : Constant  Value=Aircraft.Controls.Rud_rate_max
  Rud_rate_min : Constant  Value=Aircraft.Controls.Rud_rate_min
  Control_Surface_Const_BUS : Outport
  wires:
  Bus Creator/1 -> Control_Surface_Const_BUS/1  "Control_Surface_Const_BUS"
  Elev_pos_max/1 -> Bus Creator1/1  "Elev_pos_max_deg"
  Elev_pos_min/1 -> Bus Creator1/2  "Elev_pos_min_deg"
  Elev_rate_max/1 -> Bus Creator1/3  "Elev_rate_max_degPs"
  Elev_rate_min/1 -> Bus Creator1/4  "Elev_rate_min_degPs"
  Bus Creator1/1 -> Bus Creator/1  "Elevator_BUS"
  Ail_pos_max/1 -> Bus Creator2/1  "Ail_pos_max_deg"
  Ail_pos_min/1 -> Bus Creator2/2  "Ail_pos_min_deg"
  Ail_rate_max/1 -> Bus Creator2/3  "Ail_rate_max_degPs"
  Ail_rate_min/1 -> Bus Creator2/4  "Ail_rate_min_degPs"
  Bus Creator2/1 -> Bus Creator/2  "Aileron_BUS"
  Elev_lag/1 -> Bus Creator1/5  "Elev_lag_s"
  Ail_lag/1 -> Bus Creator2/5  "Ail_lag_s"
  Rud_pos_max/1 -> Bus Creator3/1  "Rud_pos_max_deg"
  Rud_pos_min/1 -> Bus Creator3/2  "Rud_pos_min_deg"
  Rud_rate_max/1 -> Bus Creator3/3  "Rud_rate_max_degPs"
  Rud_rate_min/1 -> Bus Creator3/4  "Rud_rate_min_degPs"
  Bus Creator3/1 -> Bus Creator/3  "Rudder_BUS"
  Rud_lag/1 -> Bus Creator3/5  "Rud_lag_s"

== system Flight_Simulation/Aircraft_Constants/Engine_Const ==
  Bus Creator : BusCreator  Inputs=8
  Engine_Ang_Mom : Constant  Value=Aircraft.Engine.Ang_Mom
  Propeler surface : Constant  Value=Aircraft.Engine.Prop_Surface
  thrust_lag : Constant  Value=Aircraft.Engine.thrust_lag
  thrust_max : Constant  Value=Aircraft.Engine.thrust_max
  thrust_min : Constant  Value=Aircraft.Engine.thrust_min
  thrust_rate_max : Constant  Value=Aircraft.Engine.thrust_rate_max
  thrust_rate_min : Constant  Value=Aircraft.Engine.thrust_rate_min
  z_eng : Constant  Value=Aircraft.Engine.z_eng
  Engine_Const_BUS : Outport
  wires:
  Engine_Ang_Mom/1 -> Bus Creator/1  "Engine_Ang_Mom_kg*m^2/s"
  Bus Creator/1 -> Engine_Const_BUS/1  "Engine_Const_BUS"
  Propeler surface/1 -> Bus Creator/2  "Propeler_S_m^2"
  thrust_max/1 -> Bus Creator/4  "thrust_max"
  thrust_min/1 -> Bus Creator/5  "thrust_min"
  thrust_rate_max/1 -> Bus Creator/6  "thrust_rate_max"
  thrust_rate_min/1 -> Bus Creator/7  "thrust_rate_min"
  thrust_lag/1 -> Bus Creator/8  "thrust_lag"
  z_eng/1 -> Bus Creator/3  "z_eng"

== system Flight_Simulation/Aircraft_Constants/Mass_Properties ==
  Bus Creator : BusCreator  Inputs=5
  J_xx : Constant  Value=Aircraft.Mass_properties.J_xx
  J_xz : Constant  Value=Aircraft.Mass_properties.J_xz
  J_yy : Constant  Value=Aircraft.Mass_properties.J_yy
  J_zz : Constant  Value=Aircraft.Mass_properties.J_zz
  Mass : Constant  Value=Aircraft.Mass_properties.Mass
  Mass_Properties_BUS : Outport
  wires:
  J_xz/1 -> Bus Creator/5  "J_xz_kg*m^2"
  J_xx/1 -> Bus Creator/2  "J_xx_kg*m^2"
  Bus Creator/1 -> Mass_Properties_BUS/1  "Mass_Properties_BUS"
  J_zz/1 -> Bus Creator/4  "J_zz_kg*m^2"
  J_yy/1 -> Bus Creator/3  "J_yy_kg*m^2"
  Mass/1 -> Bus Creator/1  "Mass_kg"

== system Flight_Simulation/Aircraft_Constants/Wing_Dimensions ==
  Bus Creator : BusCreator  Inputs=3
  MAC : Constant  Value=Aircraft.Dimensions.MAC
  WingArea : Constant  Value=Aircraft.Dimensions.WingArea
  WingSpan : Constant  Value=Aircraft.Dimensions.WingSpan
  Wing_Dimension_BUS : Outport
  wires:
  WingSpan/1 -> Bus Creator/1  "WingSpan_m"
  Bus Creator/1 -> Wing_Dimension_BUS/1  "Wing_Dimension_BUS"
  WingArea/1 -> Bus Creator/2  "WingArea_m^2"
  MAC/1 -> Bus Creator/3  "MAC_m"

== system Flight_Simulation/Control_Input/Aileron Disturbance ==
  note: no disturbance
  note: use for testing
  Step3 : Step  After=5  SampleTime=0
  Step4 : Step  Time=3  After=-5  SampleTime=0
  Step5 : Step  Time=5  After=0  SampleTime=0
  Step6 : Step  After=0  SampleTime=0
  Step7 : Step  Commented=on  Time=5  After=0.5  SampleTime=0
  Step8 : Step  Time=5  After=0  SampleTime=0
  Sum1 : Sum  Inputs=+++  InputSameDT=on  SaturateOnIntegerOverflow=on  OutDataTypeStr=Inherit: Same as first input
  Sum2 : Sum  Inputs=+++  InputSameDT=on  SaturateOnIntegerOverflow=on  OutDataTypeStr=Inherit: Same as first input
  Terminator1 : Terminator
  Terminator2 : Terminator
  Aileron_Disturbance : Outport
  wires:
  Step4/1 -> Sum1/2
  Step3/1 -> Sum1/1
  Step5/1 -> Sum1/3
  Step7/1 -> Sum2/2
  Step6/1 -> Sum2/1
  Step8/1 -> Sum2/3
  Sum2/1 -> Terminator2/1, Aileron_Disturbance/1
  Sum1/1 -> Terminator1/1

== system Flight_Simulation/Control_Input/Elevator Disturbance ==
  note: use for testing
  note: no eta disturbance
  Step3 : Step  Time=5  After=-10  SampleTime=0
  Step4 : Step  Time=10  After=+10  SampleTime=0
  Step5 : Step  Time=5  SampleTime=0
  Step6 : Step  After=0  SampleTime=0
  Step7 : Step  Commented=on  Time=5  After=0.5  SampleTime=0
  Step8 : Step  Time=5  After=0  SampleTime=0
  Sum1 : Sum  Inputs=+++  InputSameDT=on  SaturateOnIntegerOverflow=on  OutDataTypeStr=Inherit: Same as first input
  Sum2 : Sum  Inputs=+++  InputSameDT=on  SaturateOnIntegerOverflow=on  OutDataTypeStr=Inherit: Same as first input
  Terminator1 : Terminator
  Elevator_Disturbance : Outport
  wires:
  Step4/1 -> Sum1/2
  Step3/1 -> Sum1/1
  Step5/1 -> Sum1/3
  Step7/1 -> Sum2/2
  Step6/1 -> Sum2/1
  Step8/1 -> Sum2/3
  Sum2/1 -> Elevator_Disturbance/1
  Sum1/1 -> Terminator1/1

== system Flight_Simulation/Control_Input/Rudder Disturbance ==
  note: use for testing
  note: no zeta disturbance
  Step3 : Step  After=2.5  SampleTime=0
  Step4 : Step  Time=3  After=-5  SampleTime=0
  Step5 : Step  Time=5  After=2.500  SampleTime=0
  Step6 : Step  After=0  SampleTime=0
  Step7 : Step  Time=3  After=0  SampleTime=0
  Step8 : Step  Time=5  After=0  SampleTime=0
  Sum1 : Sum  Inputs=+++  InputSameDT=on  SaturateOnIntegerOverflow=on  OutDataTypeStr=Inherit: Same as first input
  Sum2 : Sum  Inputs=+++  InputSameDT=on  SaturateOnIntegerOverflow=on  OutDataTypeStr=Inherit: Same as first input
  Terminator2 : Terminator
  Rudder_Disturbance : Outport
  wires:
  Step4/1 -> Sum1/2
  Step3/1 -> Sum1/1
  Step5/1 -> Sum1/3
  Step7/1 -> Sum2/2
  Step6/1 -> Sum2/1
  Step8/1 -> Sum2/3
  Sum1/1 -> Terminator2/1
  Sum2/1 -> Rudder_Disturbance/1
